simulink model "Unit"  (R2020b)
settings: Solver=FixedStepDiscrete  StartTime=0.0  StopTime=Inf  FixedStep=0.001  RelTol=1e-3
settings Model: DataDictionary=Unit_dd.sldd  EnableAccessToBaseWorkspace=off  Creator=zhoutinglin  LastModifiedBy=zhoutinglin
settings SolverCC: ZeroCrossControl=DisableAll
settings DataIOCC: SaveOutput=off  SignalLogging=off  DSMLogging=off  SaveTime=off  ReturnWorkspaceOutputs=off
settings OptimizationCC: DefaultParameterBehavior=Inlined  EnhancedBackFolding=on  PassReuseOutputArgsAs=Individual arguments  OptimizeBlockOrder=speed  DifferentSizesBufferReuse=on  OptimizationCustomize=off  EfficientTunableParamExpr=on
settings DebuggingCC: SignalInfNanChecking=error  ReadBeforeWriteMsg=EnableAllAsWarning  WriteAfterWriteMsg=EnableAllAsWarning  WriteAfterReadMsg=EnableAllAsWarning  AlgebraicLoopMsg=error  ArtificialAlgebraicLoopMsg=error  MultiTaskDSMMsg=warning  ParameterUnderflowMsg=error  ParameterTunabilityLossMsg=error  SignalLabelMismatchMsg=error  UniqueDataStoreMsg=error  UnitsInconsistencyMsg=none  ArithmeticOperatorsInVariantConditions=warning
settings HardwareCC: ProdBitPerPointer=32  ProdBitPerSizeT=32  ProdBitPerPtrDiffT=32  ProdLargestAtomicInteger=Long  ProdLargestAtomicFloat=Double  ProdWordSize=32  ProdHWDeviceType=ARM Compatible->ARM Cortex
settings ModelReferenceCC: ModelReferenceNumInstancesAllowed=Single  PropagateSignalLabelsOutOfModel=off
settings SFSimCC: SimUseLocalCustomCode=off  SimParseCustomCode=off  MATLABDynamicMemAlloc=off  CustomCodeUndefinedFunction=UseInterfaceOnly
settings RTWCC: Description=Embedded Coder  SystemTargetFile=ert.tlc  GenCodeOnly=on  TemplateMakefile=ert_default_tmf  GenerateReport=on  RTWUseLocalCustomCode=off  IncludeHyperlinkInReport=on  LaunchReport=on  GenerateTraceInfo=on  GenerateTraceReport=on  GenerateTraceReportSl=on  GenerateTraceReportSf=on  GenerateTraceReportEml=on
settings CodeAppCC: ForceParamTrailComments=on  IgnoreCustomStorageClasses=off  OperatorAnnotations=on  SimulinkDataObjDesc=on  SFDataObjDesc=on  InsertBlockDesc=on
settings ERTTargetCC: TargetLangStandard=C99 (ISO)  GenerateSampleERTMain=on  SupportComplex=off  GenerateASAP2=on  InlinedParameterPlacement=NonHierarchical  ERTCustomFileTemplate=example_file_process.tlc  MemSecPackage=Simulink  MemSecDataIO=MemVolatile  MemSecDataParameters=MemConstVolatile
settings ConfigComp: CovScope=ReferencedModels  CovIncludeTopModel=off  CovMetricSettings=dcmwe

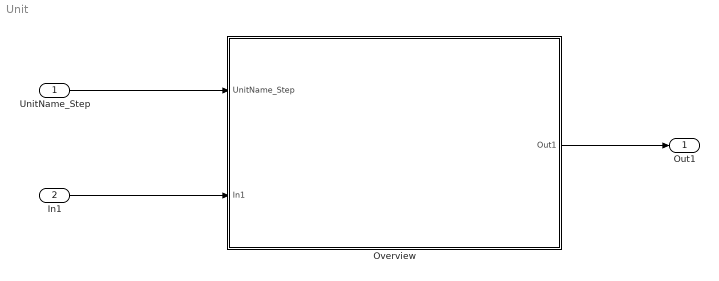
== system Unit ==
  UnitName_Step : Inport  OutputFunctionCall=on
  In1 : Inport  Port=2
  Overview : Subsystem
  Out1 : Outport  VectorParamsAs1DForOutWhenUnconnected=off
  wires:
  UnitName_Step/1 -> Overview/1(UnitName_Step)
  In1/1 -> Overview/2(In1)
  Overview/1(Out1) -> Out1/1

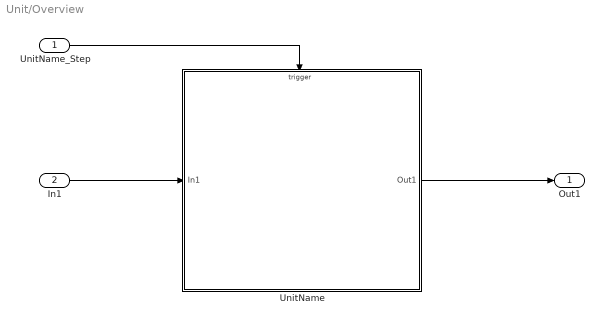
== system Unit/Overview ==
  UnitName_Step : Inport
  In1 : Inport  Port=2
  UnitName : Subsystem  TreatAsAtomicUnit=on
  Out1 : Outport  VectorParamsAs1DForOutWhenUnconnected=off
  wires:
  UnitName_Step/1 -> UnitName/Trigger
  In1/1 -> UnitName/1(In1)
  UnitName/1(Out1) -> Out1/1

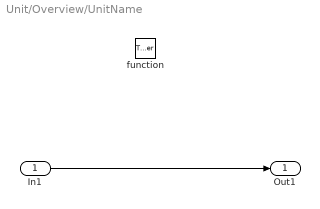
== system Unit/Overview/UnitName ==
  In1 : Inport
  function : TriggerPort  TriggerType=function-call  VariantControl=Variant
  Out1 : Outport  VectorParamsAs1DForOutWhenUnconnected=off
  wires:
  In1/1 -> Out1/1
